simulink model "cartPole"  (R2016a)
settings: Solver=ode45  StartTime=0.0  StopTime=20  FixedStep=4/149  MaxStep=0.0001  RelTol=1e-3
values from neighbouring files (symbols this model uses):
  dtheta_initial = 0    [dynamicEquation_cartPole.m]
  dx_initial = 0    [dynamicEquation_cartPole.m]
  feedbackGain = -place(A, B, p)    [dynamicEquation_cartPole.m]
  gravity = g    (= 9.81)    [dynamicEquation_cartPole.m]
  l_pend = l    (= 1)    [dynamicEquation_cartPole.m]
  m_b = m_body    (= 0.1)    [dynamicEquation_cartPole.m]
  m_c = m_cart    (= 1)    [dynamicEquation_cartPole.m]
  theta_initial = 1    [dynamicEquation_cartPole.m]
  x_initial = 0    [dynamicEquation_cartPole.m]
undefined symbols (not defined in the file or in its folder): Energy_desired, input, k_E, kd, kp
settings Model: Creator=Puneet  LastModifiedBy=Puneet
settings GRTTargetCC: GeneratePreprocessorConditionals=Use local settings

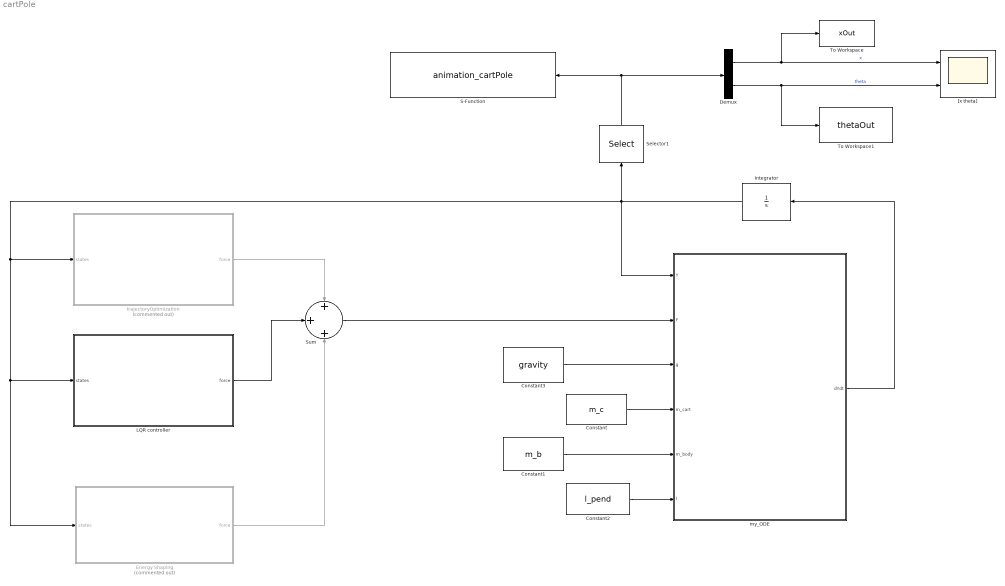
== system cartPole ==
  Constant : Constant  Value=m_c
  Constant1 : Constant  Value=m_b
  Constant2 : Constant  Value=l_pend
  Constant3 : Constant  Value=gravity
  Demux : Demux  Outputs=2
  Energy Shaping : Subsystem  Commented=on
  Integrator : Integrator  InitialCondition=[x_initial, dx_initial, theta_initial, dtheta_initial]
  LQR controller : Subsystem
  S-Function : S-Function  FunctionName=animation_cartPole  Parameters=0.01  SFunctionDeploymentMode=off  EnableBusSupport=off
  Selector1 : Selector  InputPortWidth=4  IndexOptions=Index vector (dialog)  Indices=[1 3]  OutputSizes=1
  Sum : Sum  Inputs=+++
  To Workspace : ToWorkspace  VariableName=xOut  SaveFormat=Timeseries  SampleTime=-1
  To Workspace1 : ToWorkspace  VariableName=thetaOut  SaveFormat=Timeseries  SampleTime=-1
  "[x theta]" : Scope  NumInputPorts=2
  my_ODE : MATLAB Function  TreatAsAtomicUnit=on
  trajectoryOptimization : Subsystem  Commented=on
  wires:
  Constant/1 -> my_ODE/4(m_cart)
  Constant1/1 -> my_ODE/5(m_body)
  Constant2/1 -> my_ODE/6(l)
  Constant3/1 -> my_ODE/3(g)
  Selector1/1 -> Demux/1, S-Function/1
  Demux/1 -> To Workspace/1, "[x theta]"/1  "x"
  Demux/2 -> To Workspace1/1, "[x theta]"/2  "theta"
  my_ODE/1(dYdt) -> Integrator/1
  Integrator/1 -> my_ODE/1(Y), Energy Shaping/1(states), LQR controller/1(states), trajectoryOptimization/1(states), Selector1/1
  trajectoryOptimization/1(force) -> Sum/1
  LQR controller/1(force) -> Sum/2
  Sum/1 -> my_ODE/2(F)
  Energy Shaping/1(force) -> Sum/3

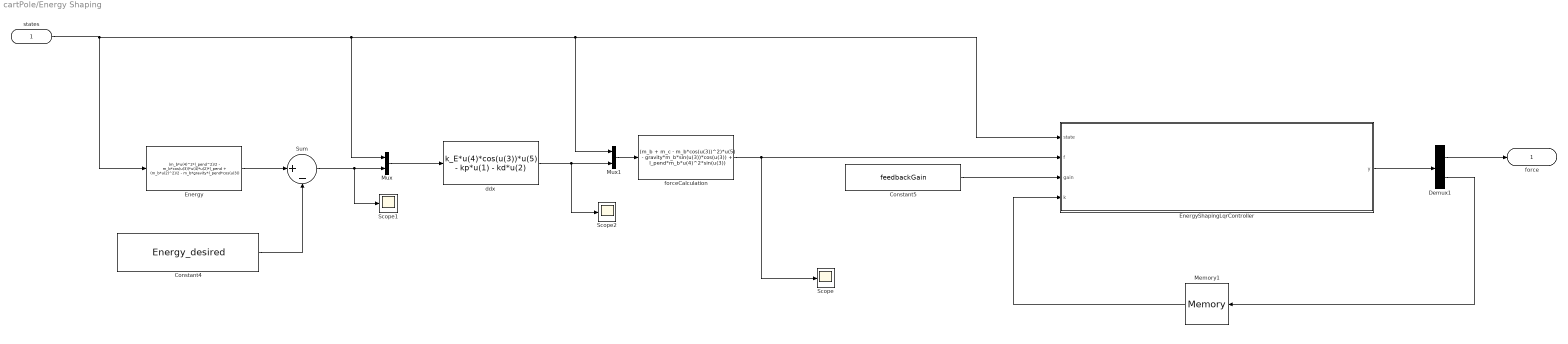
== system cartPole/Energy Shaping ==
  states : Inport
  Constant4 : Constant  Value=Energy_desired
  Constant5 : Constant  Value=feedbackGain
  Demux1 : Demux  Outputs=2
  Energy : Fcn  Expr=|
      | (m_b*u(4)^2*l_pend^2)/2 - m_b*cos(u(3))*u(4)*u(2)*l_pend 
      | + (m_b*u(2)^2)/2 - m_b*gravity*l_pend*cos(u(3))
  EnergyShapingLqrController : MATLAB Function  TreatAsAtomicUnit=on
  Memory1 : Memory  X0=1
  Mux : Mux  Inputs=2
  Mux1 : Mux  Inputs=2
  Scope : Scope
  Scope1 : Scope
  Scope2 : Scope
  Sum : Sum  Inputs=|+-
  ddx : Fcn  Expr=k_E*u(4)*cos(u(3))*u(5) - kp*u(1) - kd*u(2)
  forceCalculation : Fcn  Expr=(m_b + m_c - m_b*cos(u(3))^2)*u(5) - gravity*m_b*sin(u(3))*cos(u(3)) + l_pend*m_b*u(4)^2*sin(u(3))
  force : Outport
  wires:
  Constant4/1 -> Sum/2
  Energy/1 -> Sum/1
  Sum/1 -> Scope1/1, Mux/2
  Mux/1 -> ddx/1
  ddx/1 -> Scope2/1, Mux1/2
  Mux1/1 -> forceCalculation/1
  Memory1/1 -> EnergyShapingLqrController/4(k)
  EnergyShapingLqrController/1(y) -> Demux1/1
  Demux1/2 -> Memory1/1
  Constant5/1 -> EnergyShapingLqrController/3(gain)
  forceCalculation/1 -> EnergyShapingLqrController/2(f), Scope/1
  states/1 -> EnergyShapingLqrController/1(state), Mux1/1, Mux/1, Energy/1
  Demux1/1 -> force/1

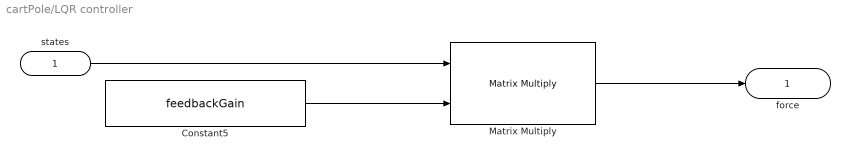
== system cartPole/LQR controller ==
  states : Inport
  Constant5 : Constant  Value=feedbackGain
  Matrix Multiply : Product  Multiplication=Matrix(*)
  force : Outport
  wires:
  Constant5/1 -> Matrix Multiply/2
  states/1 -> Matrix Multiply/1
  Matrix Multiply/1 -> force/1

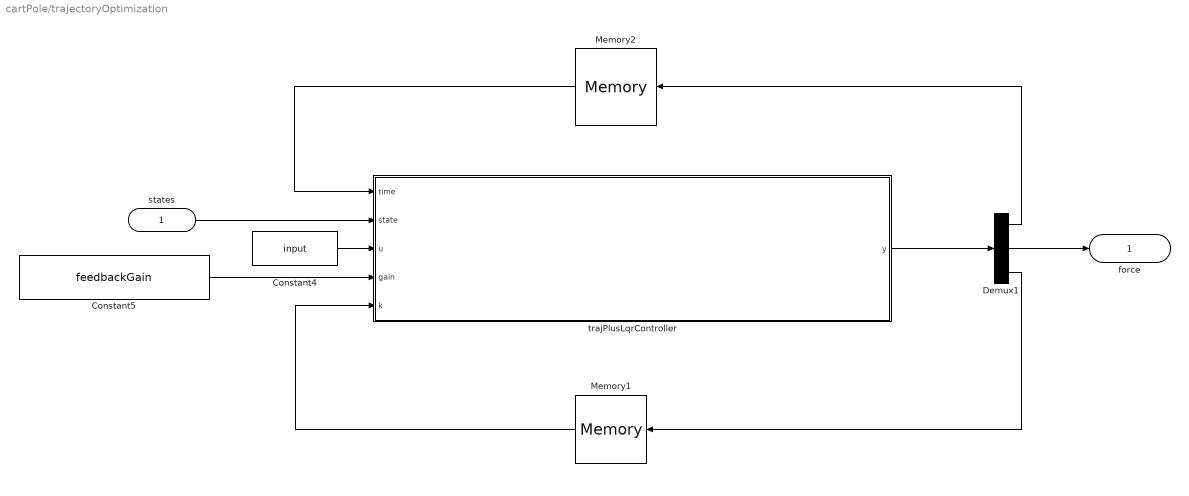
== system cartPole/trajectoryOptimization ==
  states : Inport
  Constant4 : Constant  Value=input
  Constant5 : Constant  Value=feedbackGain
  Demux1 : Demux  Outputs=3
  Memory1 : Memory  X0=1
  Memory2 : Memory
  trajPlusLqrController : MATLAB Function  TreatAsAtomicUnit=on
  force : Outport
  wires:
  Memory1/1 -> trajPlusLqrController/5(k)
  trajPlusLqrController/1(y) -> Demux1/1
  Demux1/1 -> Memory2/1
  Demux1/2 -> force/1
  Memory2/1 -> trajPlusLqrController/1(time)
  Demux1/3 -> Memory1/1
  Constant5/1 -> trajPlusLqrController/4(gain)
  states/1 -> trajPlusLqrController/2(state)
  Constant4/1 -> trajPlusLqrController/3(u)

== matlab function cartPole/trajectoryOptimization/trajPlusLqrController ==
  data: time input; state input; u input; gain input; k input; y output
function y = trajPlusLqrController(time, state, u, gain, k)
%#codegen
time = time + 0.2;
coder.extrinsic('wrapToPi');
state(3) = wrapToPi(state(3));
if (abs(state(3)-0)<0.2)
    k=2;
% elseif (state(3)>pi && (2*pi - state(3))<0.2)
%     k=2;
end

if (k==2)
    
    force = gain(1)*state(1)+ gain(2)*state(2) + gain(3)*state(3) + gain(4)*state(4);
else
%     time
    force = u(floor(time*4/149)+1);
end

y = [time, force, k];

== matlab function cartPole/my_ODE ==
  data: dYdt output; Y input; F input; g input; m_cart input; m_body input; l input
function dYdt = my_ODE(Y,F,g,m_cart,m_body,l)
%#codegen

%    This function was generated by the Symbolic Math Toolbox version 7.0.
%    18-Feb-2017 18:54:45

t3 = Y(3);
t2 = cos(t3);
t4 = sin(t3);
t5 = Y(4);
t6 = t2.^2;
t7 = m_body+m_cart-m_body.*t6;
t8 = 1.0./t7;
t9 = t5.^2;
dYdt = [Y(2);t8.*(F+g.*m_body.*t2.*t4-l.*m_body.*t4.*t9);t5;(t8.*(F.*t2+g.*m_body.*t4+g.*m_cart.*t4-l.*m_body.*t2.*t4.*t9))./l];

== matlab function cartPole/Energy Shaping/EnergyShapingLqrController ==
  data: state input; f input; gain input; k input; y output
function y = EnergyShapingLqrController(state, f, gain, k)
%#codegen

coder.extrinsic('wrapToPi');
% state(3) = wrapToPi(state(3));
if (abs(state(3)-0)<0.2)
    k=2;
% elseif (state(3)>pi && (2*pi - state(3))<0.2)
%     k=2;
end

if (k==2)
    
    force = gain(1)*state(1)+ gain(2)*state(2) + gain(3)*state(3) + gain(4)*state(4);
else
%     time
    force = f;
end

y = [force, k];
